simulink model "Drone2_simulink"  (R2024a)
settings: Solver=ode1be  StartTime=0.0  StopTime=1000  FixedStep=0.001  MaxStep=0.001  MinStep=0.00095  RelTol=1e-3
PreLoadFcn:
  | Drone_data;
model workspace: external: MATLAB File C:\Users\admin\OneDrive - Indian Institute of Technology Jodhpur\IIT JODHPUR\Research Work\Amphibious Drone\MATLAB_CODE\2025\New_Drone\Drone_1\Drone1_simulink_DataFile.m (data not in the file)
undefined symbols (not defined in the file): Environment, Newton, Raphson, Vehicle, X, Y, Z
libraries: sm_lib x1684, nesl_utility x63, slpidlib x25, eeGeneralControl x6, matrix_library x3, rllib x2, simulink x2, fl_lib x1, sharedutil x1, SignalEditorBlockLib x1
(part 15 of 17)

== system Drone2_simulink/Physical_system/Drone_Assembly/Cylinder_Assembly/Frontcap/Nut on Cap/Nutwasher_subsystem5 ==
  m3nut1 : sm_lib/Body Elements/File Solid  ExtGeomFileName=socket head cap screw_isM3.STL  UnitType=Custom  ExtGeomFileUnits=mm  StepReaderType=HEX  ExportConvexHullGeometry=off  InertiaType=CalculateFromGeometry  BasedOnType=Density  Density=7800  DensityUnits=kg/m^3  Mass=1  MassUnits=kg  CenterOfMass=[0 0 0]  CenterOfMassUnits=m  MomentsOfInertia=[1 1 1]  MomentsOfInertiaUnits=kg*m^2  ProductsOfInertia=[0 0 0]  ProductsOfInertiaUnits=kg*m^2  GraphicType=FromGeometry  MarkerShape=Sphere  MarkerSize=10  GraphicVisPropType=SimpleVisualProperties  GraphicDiffuseColor=[0.5 0.5 0.5]  GraphicOpacity=1  GraphicSpecularColor=[0.5 0.5 0.5 1.0]  GraphicAmbientColor=[0.15 0.15 0.15 1.0]  GraphicEmissiveColor=[0.0 0.0 0.0 1.0]  GraphicShininess=75  DoExposeReferenceFrame=off  SerializedFrames=<Frames><Frame><Id>Frame1</Id><Value><Name>F1</Name><Origin><Source>CenterOfMassFrame</Source><FeatureName></FeatureName></Origin><PrimaryAxis><DefinedDirection>+Z</DefinedDirection><Source>ReferenceFrame</Source><SourceDirection>-X</SourceDirection><FeatureName></FeatureName></PrimaryAxis><SecondaryAxis><DefinedDirection>+X</DefinedDirection><Source>ReferenceFrame</Source><SourceDirection>+Y</SourceDirection><FeatureName></FeatureName></SecondaryAxis></Value></Frame></Frames>
  m3washer1 : sm_lib/Body Elements/File Solid  ExtGeomFileName=plain washer (type a)_isM3.STL  UnitType=Custom  ExtGeomFileUnits=mm  StepReaderType=HEX  ExportConvexHullGeometry=off  InertiaType=CalculateFromGeometry  BasedOnType=Density  Density=7800  DensityUnits=kg/m^3  Mass=1  MassUnits=kg  CenterOfMass=[0 0 0]  CenterOfMassUnits=m  MomentsOfInertia=[1 1 1]  MomentsOfInertiaUnits=kg*m^2  ProductsOfInertia=[0 0 0]  ProductsOfInertiaUnits=kg*m^2  GraphicType=FromGeometry  MarkerShape=Sphere  MarkerSize=10  GraphicVisPropType=SimpleVisualProperties  GraphicDiffuseColor=[0.5 0.5 0.5]  GraphicOpacity=1  GraphicSpecularColor=[0.5 0.5 0.5 1.0]  GraphicAmbientColor=[0.15 0.15 0.15 1.0]  GraphicEmissiveColor=[0.0 0.0 0.0 1.0]  GraphicShininess=75  DoExposeReferenceFrame=off  SerializedFrames=<Frames><Frame><Id>Frame1</Id><Value><Name>F1</Name><Origin><Source>CenterOfMassFrame</Source><FeatureName></FeatureName></Origin><PrimaryAxis><DefinedDirection>+Z</DefinedDirection><Source>ReferenceFrame</Source><SourceDirection>+Y</SourceDirection><FeatureName></FeatureName></PrimaryAxis><SecondaryAxis><DefinedDirection>+X</DefinedDirection><Source>ReferenceFrame</Source><SourceDirection>+X</SourceDirection><FeatureName></FeatureName></SecondaryAxis></Value></Frame></Frames>
  ofsetfornut : sm_lib/Frames and Transforms/Rigid Transform  RotationMethod=None  FollAlignAxisA=+X  BaseAlignAxisA=+Y  FollAlignAxisB=+Y  BaseAlignAxisB=+Z  RotationStandardAxis=+Z  RotationAngle=180  RotationAngleUnits=deg  RotationArbitraryAxis=[0 0 1]  RotationSequenceAxes=FollowerAxes  RotationSequence=XYX  RotationSequenceAngles=[0 0 0]  RotationSequenceAnglesUnits=deg  RotationMatrix=[1 0 0;0 1 0;0 0 1]  Quaternion=[1 0 0 0]  TranslationMethod=Cartesian  TranslationCartesianOffset=[0 0 -0.0043]  TranslationCartesianOffsetUnits=m  TranslationStandardAxis=+Z  TranslationStandardOffset=0  TranslationStandardOffsetUnits=m  TranslationROffset=0  TranslationROffsetUnits=m  TranslationThetaOffset=0  TranslationThetaOffsetUnits=deg  TranslationZOffset=0  TranslationZOffsetUnits=m
  washercentre to washer1 : sm_lib/Frames and Transforms/Rigid Transform  RotationMethod=None  FollAlignAxisA=+X  BaseAlignAxisA=+Z  FollAlignAxisB=+Y  BaseAlignAxisB=+Y  RotationStandardAxis=+Z  RotationAngle=180  RotationAngleUnits=deg  RotationArbitraryAxis=[0 0 1]  RotationSequenceAxes=FollowerAxes  RotationSequence=XYX  RotationSequenceAngles=[0 0 0]  RotationSequenceAnglesUnits=deg  RotationMatrix=[1 0 0;0 1 0;0 0 1]  Quaternion=[1 0 0 0]  TranslationMethod=Cylindrical  TranslationCartesianOffset=[0.227 0 0]  TranslationCartesianOffsetUnits=m  TranslationStandardAxis=+Z  TranslationStandardOffset=0  TranslationStandardOffsetUnits=m  TranslationROffset=0.0675  TranslationROffsetUnits=m  TranslationThetaOffset=theta  TranslationThetaOffsetUnits=deg  TranslationZOffset=0.00025  TranslationZOffsetUnits=m
  fromcenter : PMIOPort  Side=Left
  connections:
  m3washer1/LConn1 -- washercentre to washer1/RConn1 -- ofsetfornut/LConn1
  ofsetfornut/RConn1 -- m3nut1/LConn1
  fromcenter/RConn1 -- washercentre to washer1/LConn1

== system Drone2_simulink/Physical_system/Drone_Assembly/Cylinder_Assembly/Frontcap/Nut on Cap/Nutwasher_subsystem6 ==
  m3nut1 : sm_lib/Body Elements/File Solid  ExtGeomFileName=socket head cap screw_isM3.STL  UnitType=Custom  ExtGeomFileUnits=mm  StepReaderType=HEX  ExportConvexHullGeometry=off  InertiaType=CalculateFromGeometry  BasedOnType=Density  Density=7800  DensityUnits=kg/m^3  Mass=1  MassUnits=kg  CenterOfMass=[0 0 0]  CenterOfMassUnits=m  MomentsOfInertia=[1 1 1]  MomentsOfInertiaUnits=kg*m^2  ProductsOfInertia=[0 0 0]  ProductsOfInertiaUnits=kg*m^2  GraphicType=FromGeometry  MarkerShape=Sphere  MarkerSize=10  GraphicVisPropType=SimpleVisualProperties  GraphicDiffuseColor=[0.5 0.5 0.5]  GraphicOpacity=1  GraphicSpecularColor=[0.5 0.5 0.5 1.0]  GraphicAmbientColor=[0.15 0.15 0.15 1.0]  GraphicEmissiveColor=[0.0 0.0 0.0 1.0]  GraphicShininess=75  DoExposeReferenceFrame=off  SerializedFrames=<Frames><Frame><Id>Frame1</Id><Value><Name>F1</Name><Origin><Source>CenterOfMassFrame</Source><FeatureName></FeatureName></Origin><PrimaryAxis><DefinedDirection>+Z</DefinedDirection><Source>ReferenceFrame</Source><SourceDirection>-X</SourceDirection><FeatureName></FeatureName></PrimaryAxis><SecondaryAxis><DefinedDirection>+X</DefinedDirection><Source>ReferenceFrame</Source><SourceDirection>+Y</SourceDirection><FeatureName></FeatureName></SecondaryAxis></Value></Frame></Frames>
  m3washer1 : sm_lib/Body Elements/File Solid  ExtGeomFileName=plain washer (type a)_isM3.STL  UnitType=Custom  ExtGeomFileUnits=mm  StepReaderType=HEX  ExportConvexHullGeometry=off  InertiaType=CalculateFromGeometry  BasedOnType=Density  Density=7800  DensityUnits=kg/m^3  Mass=1  MassUnits=kg  CenterOfMass=[0 0 0]  CenterOfMassUnits=m  MomentsOfInertia=[1 1 1]  MomentsOfInertiaUnits=kg*m^2  ProductsOfInertia=[0 0 0]  ProductsOfInertiaUnits=kg*m^2  GraphicType=FromGeometry  MarkerShape=Sphere  MarkerSize=10  GraphicVisPropType=SimpleVisualProperties  GraphicDiffuseColor=[0.5 0.5 0.5]  GraphicOpacity=1  GraphicSpecularColor=[0.5 0.5 0.5 1.0]  GraphicAmbientColor=[0.15 0.15 0.15 1.0]  GraphicEmissiveColor=[0.0 0.0 0.0 1.0]  GraphicShininess=75  DoExposeReferenceFrame=off  SerializedFrames=<Frames><Frame><Id>Frame1</Id><Value><Name>F1</Name><Origin><Source>CenterOfMassFrame</Source><FeatureName></FeatureName></Origin><PrimaryAxis><DefinedDirection>+Z</DefinedDirection><Source>ReferenceFrame</Source><SourceDirection>+Y</SourceDirection><FeatureName></FeatureName></PrimaryAxis><SecondaryAxis><DefinedDirection>+X</DefinedDirection><Source>ReferenceFrame</Source><SourceDirection>+X</SourceDirection><FeatureName></FeatureName></SecondaryAxis></Value></Frame></Frames>
  ofsetfornut : sm_lib/Frames and Transforms/Rigid Transform  RotationMethod=None  FollAlignAxisA=+X  BaseAlignAxisA=+Y  FollAlignAxisB=+Y  BaseAlignAxisB=+Z  RotationStandardAxis=+Z  RotationAngle=180  RotationAngleUnits=deg  RotationArbitraryAxis=[0 0 1]  RotationSequenceAxes=FollowerAxes  RotationSequence=XYX  RotationSequenceAngles=[0 0 0]  RotationSequenceAnglesUnits=deg  RotationMatrix=[1 0 0;0 1 0;0 0 1]  Quaternion=[1 0 0 0]  TranslationMethod=Cartesian  TranslationCartesianOffset=[0 0 -0.0043]  TranslationCartesianOffsetUnits=m  TranslationStandardAxis=+Z  TranslationStandardOffset=0  TranslationStandardOffsetUnits=m  TranslationROffset=0  TranslationROffsetUnits=m  TranslationThetaOffset=0  TranslationThetaOffsetUnits=deg  TranslationZOffset=0  TranslationZOffsetUnits=m
  washercentre to washer1 : sm_lib/Frames and Transforms/Rigid Transform  RotationMethod=None  FollAlignAxisA=+X  BaseAlignAxisA=+Z  FollAlignAxisB=+Y  BaseAlignAxisB=+Y  RotationStandardAxis=+Z  RotationAngle=180  RotationAngleUnits=deg  RotationArbitraryAxis=[0 0 1]  RotationSequenceAxes=FollowerAxes  RotationSequence=XYX  RotationSequenceAngles=[0 0 0]  RotationSequenceAnglesUnits=deg  RotationMatrix=[1 0 0;0 1 0;0 0 1]  Quaternion=[1 0 0 0]  TranslationMethod=Cylindrical  TranslationCartesianOffset=[0.227 0 0]  TranslationCartesianOffsetUnits=m  TranslationStandardAxis=+Z  TranslationStandardOffset=0  TranslationStandardOffsetUnits=m  TranslationROffset=0.0675  TranslationROffsetUnits=m  TranslationThetaOffset=theta  TranslationThetaOffsetUnits=deg  TranslationZOffset=0.00025  TranslationZOffsetUnits=m
  fromcenter : PMIOPort  Side=Left
  connections:
  m3washer1/LConn1 -- washercentre to washer1/RConn1 -- ofsetfornut/LConn1
  ofsetfornut/RConn1 -- m3nut1/LConn1
  fromcenter/RConn1 -- washercentre to washer1/LConn1

== system Drone2_simulink/Physical_system/Drone_Assembly/Cylinder_Assembly/Frontcap/Nut on Cap/Nutwasher_subsystem7 ==
  m3nut1 : sm_lib/Body Elements/File Solid  ExtGeomFileName=socket head cap screw_isM3.STL  UnitType=Custom  ExtGeomFileUnits=mm  StepReaderType=HEX  ExportConvexHullGeometry=off  InertiaType=CalculateFromGeometry  BasedOnType=Density  Density=7800  DensityUnits=kg/m^3  Mass=1  MassUnits=kg  CenterOfMass=[0 0 0]  CenterOfMassUnits=m  MomentsOfInertia=[1 1 1]  MomentsOfInertiaUnits=kg*m^2  ProductsOfInertia=[0 0 0]  ProductsOfInertiaUnits=kg*m^2  GraphicType=FromGeometry  MarkerShape=Sphere  MarkerSize=10  GraphicVisPropType=SimpleVisualProperties  GraphicDiffuseColor=[0.5 0.5 0.5]  GraphicOpacity=1  GraphicSpecularColor=[0.5 0.5 0.5 1.0]  GraphicAmbientColor=[0.15 0.15 0.15 1.0]  GraphicEmissiveColor=[0.0 0.0 0.0 1.0]  GraphicShininess=75  DoExposeReferenceFrame=off  SerializedFrames=<Frames><Frame><Id>Frame1</Id><Value><Name>F1</Name><Origin><Source>CenterOfMassFrame</Source><FeatureName></FeatureName></Origin><PrimaryAxis><DefinedDirection>+Z</DefinedDirection><Source>ReferenceFrame</Source><SourceDirection>-X</SourceDirection><FeatureName></FeatureName></PrimaryAxis><SecondaryAxis><DefinedDirection>+X</DefinedDirection><Source>ReferenceFrame</Source><SourceDirection>+Y</SourceDirection><FeatureName></FeatureName></SecondaryAxis></Value></Frame></Frames>
  m3washer1 : sm_lib/Body Elements/File Solid  ExtGeomFileName=plain washer (type a)_isM3.STL  UnitType=Custom  ExtGeomFileUnits=mm  StepReaderType=HEX  ExportConvexHullGeometry=off  InertiaType=CalculateFromGeometry  BasedOnType=Density  Density=7800  DensityUnits=kg/m^3  Mass=1  MassUnits=kg  CenterOfMass=[0 0 0]  CenterOfMassUnits=m  MomentsOfInertia=[1 1 1]  MomentsOfInertiaUnits=kg*m^2  ProductsOfInertia=[0 0 0]  ProductsOfInertiaUnits=kg*m^2  GraphicType=FromGeometry  MarkerShape=Sphere  MarkerSize=10  GraphicVisPropType=SimpleVisualProperties  GraphicDiffuseColor=[0.5 0.5 0.5]  GraphicOpacity=1  GraphicSpecularColor=[0.5 0.5 0.5 1.0]  GraphicAmbientColor=[0.15 0.15 0.15 1.0]  GraphicEmissiveColor=[0.0 0.0 0.0 1.0]  GraphicShininess=75  DoExposeReferenceFrame=off  SerializedFrames=<Frames><Frame><Id>Frame1</Id><Value><Name>F1</Name><Origin><Source>CenterOfMassFrame</Source><FeatureName></FeatureName></Origin><PrimaryAxis><DefinedDirection>+Z</DefinedDirection><Source>ReferenceFrame</Source><SourceDirection>+Y</SourceDirection><FeatureName></FeatureName></PrimaryAxis><SecondaryAxis><DefinedDirection>+X</DefinedDirection><Source>ReferenceFrame</Source><SourceDirection>+X</SourceDirection><FeatureName></FeatureName></SecondaryAxis></Value></Frame></Frames>
  ofsetfornut : sm_lib/Frames and Transforms/Rigid Transform  RotationMethod=None  FollAlignAxisA=+X  BaseAlignAxisA=+Y  FollAlignAxisB=+Y  BaseAlignAxisB=+Z  RotationStandardAxis=+Z  RotationAngle=180  RotationAngleUnits=deg  RotationArbitraryAxis=[0 0 1]  RotationSequenceAxes=FollowerAxes  RotationSequence=XYX  RotationSequenceAngles=[0 0 0]  RotationSequenceAnglesUnits=deg  RotationMatrix=[1 0 0;0 1 0;0 0 1]  Quaternion=[1 0 0 0]  TranslationMethod=Cartesian  TranslationCartesianOffset=[0 0 -0.0043]  TranslationCartesianOffsetUnits=m  TranslationStandardAxis=+Z  TranslationStandardOffset=0  TranslationStandardOffsetUnits=m  TranslationROffset=0  TranslationROffsetUnits=m  TranslationThetaOffset=0  TranslationThetaOffsetUnits=deg  TranslationZOffset=0  TranslationZOffsetUnits=m
  washercentre to washer1 : sm_lib/Frames and Transforms/Rigid Transform  RotationMethod=None  FollAlignAxisA=+X  BaseAlignAxisA=+Z  FollAlignAxisB=+Y  BaseAlignAxisB=+Y  RotationStandardAxis=+Z  RotationAngle=180  RotationAngleUnits=deg  RotationArbitraryAxis=[0 0 1]  RotationSequenceAxes=FollowerAxes  RotationSequence=XYX  RotationSequenceAngles=[0 0 0]  RotationSequenceAnglesUnits=deg  RotationMatrix=[1 0 0;0 1 0;0 0 1]  Quaternion=[1 0 0 0]  TranslationMethod=Cylindrical  TranslationCartesianOffset=[0.227 0 0]  TranslationCartesianOffsetUnits=m  TranslationStandardAxis=+Z  TranslationStandardOffset=0  TranslationStandardOffsetUnits=m  TranslationROffset=0.0675  TranslationROffsetUnits=m  TranslationThetaOffset=theta  TranslationThetaOffsetUnits=deg  TranslationZOffset=0.00025  TranslationZOffsetUnits=m
  fromcenter : PMIOPort  Side=Left
  connections:
  m3washer1/LConn1 -- washercentre to washer1/RConn1 -- ofsetfornut/LConn1
  ofsetfornut/RConn1 -- m3nut1/LConn1
  fromcenter/RConn1 -- washercentre to washer1/LConn1

== matlab function Drone2_simulink/Controller/Aerial_control/Aerial Control ==
  data: Thrust input; FRF output; TRF output; Roll input; Pitch input; Yaw input; FRB output; TRB output; FLF output; TLF output; FLB output; TLB output; k parameter; Zd input; Z input; ez input; ez_dot input; er input; er_dot input; ep input; ep_dot input; eyaw input; eyaw_dot input; Max_thrust parameter; Min_torque parameter; Max_torque parameter; Min_Dthrust parameter; dt parameter; EZ_DB parameter; ER_DB parameter; EP_DB parameter; Eyaw_DB parameter
function [FRF,TRF, FRB, TRB,FLF,TLF, FLB,TLB] = fcn(Thrust,Roll,Pitch,Yaw,k,Zd,Z,ez,ez_dot,er,er_dot,ep,ep_dot,eyaw,eyaw_dot, Max_thrust, Min_torque, Max_torque,Min_Dthrust,dt,EZ_DB, ER_DB, EP_DB, Eyaw_DB)
A  = [1 1 1 1;0.276 0.276 -0.276 -0.276;-0.1575 0.1825 0.1825 -0.1575;-k k -k k];
if Zd<=0 && Z >=0
   [FRF, FRB,FLF, FLB] = deal(0);
   [TRF, TRB,TLF,TLB] = deal(0);
    return
elseif Zd<=0 && Z<0
    [FRF,TRF, FRB, TRB,FLF,TLF, FLB,TLB] = deal(0);
    return
elseif Z <=-0.15
    [FRF,TRF, FRB, TRB,FLF,TLF, FLB,TLB] = deal(0);
    return
end


Force = A\[Thrust;Roll;Pitch;Yaw];



%% Adaptive Part
K_TRIM = 0.002;
K_RATE = 0.005;

adapt_gateZ = 1.0 / (1.0 + K_RATE*abs(ez_dot));     % suppress when moving fast
if abs(ez) < EZ_DB
    adapt_gateZ = 0.25 * adapt_gateZ;                 % slower inside small band0.2
end
dSum_trimZ = K_TRIM * ez * adapt_gateZ;  

adapt_gateR = 1.0 / (1.0 + K_RATE*abs(er_dot));     % suppress when moving fast
if abs(er) < ER_DB
    adapt_gateR = 0.25* adapt_gateR;                 % slower inside small band0.2
end
dSum_trimR = K_TRIM * ez * adapt_gateR; 

adapt_gateP = 1.0 / (1.0 + K_RATE*abs(ep_dot));     % suppress when moving fast
if abs(ep) < EP_DB
    adapt_gateP = 0.25 * adapt_gateP;                 % slower inside small band0.2
end
dSum_trimP = K_TRIM * ez * adapt_gateP;  

adapt_gateY = 1.0 / (1.0 + K_RATE*abs(eyaw_dot));     % suppress when moving fast
if abs(eyaw) < Eyaw_DB
    adapt_gateY = 0.25 * adapt_gateY;                 % slower inside small band0.2
end
dSum_trimY = K_TRIM * ez * adapt_gateY;  

FLF = Force(1);%+dSum_trimZ*dt+dSum_trimR*dt-dSum_trimP*dt ;
FLB = Force(2);%+dSum_trimZ*dt+dSum_trimR*dt+dSum_trimP*dt;
FRB = Force(3);%+dSum_trimZ*dt-dSum_trimR*dt+dSum_trimP*dt;
FRF = Force(4);%+dSum_trimZ*dt-dSum_trimR*dt-dSum_trimP*dt;
TRF = k*FRF;%+dSum_trimY;
TRB = k*FRB;%-dSum_trimY;
TLF = k*FLF;%-dSum_trimY;
TLB = k*FLB;%+dSum_trimY;

FLF = clamp(FLF,Min_Dthrust,Max_thrust);
FLB = clamp(FLB,Min_Dthrust,Max_thrust);
FRF = clamp(FRF,Min_Dthrust,Max_thrust);
FRB = clamp(FRB,Min_Dthrust,Max_thrust);

TLF = clamp(TLF,Min_torque,Max_torque);
TLB = clamp(TLB,Min_torque,Max_torque);
TRF = clamp(TRF,Min_torque,Max_torque);
TRB = clamp(TRB,Min_torque,Max_torque);
end


function y = clamp(x, xmin, xmax)
    y = min(max(x, xmin), xmax);
end

== matlab function Drone2_simulink/Controller/RL System/MATLAB Function2 ==
  data: Obsevation input; reward output; Desired input; feedback input; Const parameter
%% reward Function
function reward = rewardFunction(Obsevation,Desired,feedback, Const)
% Target depth and pitch
depth = Observation(1);
depthRate = Obsevation(2);
pitch= Obsevation(3);
pitchRate = Obsevation(4);
Fs1pos = Obsevation(5);
Fs2pos = Obsevation(6);
Fs1vel = Obsevation(7);
Fs2vel = Obsevation(8);
Bspos = Obsevation(9);
Bsvel = Obsevation(10);
A = const;
depth_ref = Desired(1);
pitch_ref = Desired(2);



depth_error = depth - depth_ref;
pitch_error = pitch - pitch_ref;


reward = - (5 * depth_error^2 + 2 * pitch_error^2 + 0.5 * depthRate^2 + 0.5 * pitchRate^2);
end

== matlab function Drone2_simulink/Controller/RL System/MATLAB Function3 ==
  data: Observation input; reward output; Desired input; MaxVel parameter; MaxPose parameter; MinPose parameter; Delta parameter; K parameter
%% reward Function
function reward = rewardFunction(Observation,Desired, MaxVel, MaxPose, MinPose, Delta, K)
% Target depth and pitch
depth = Observation(1);
depthRate = Observation(2);
pitch= Observation(3);
pitchRate = Observation(4);
Fs1pos = Observation(5);
Fs2pos = Observation(6);
Fs1vel = Observation(7);
Fs2vel = Observation(8);
Bspos = Observation(9);
Bsvel = Observation(10);


Syring1Reward = syringeRewardSigmoid(Fs1pos,Fs1vel,MinPose,MaxPose,Delta,MaxVel,K);
Syring2Reward = syringeRewardSigmoid(Fs2pos,Fs2vel,MinPose,MaxPose,Delta,MaxVel,K);
Syring3Reward = syringeRewardSigmoid(Bspos,Bsvel,MinPose,MaxPose,Delta,MaxVel,K);


depth_ref = Desired(1);
pitch_ref = Desired(2);



depth_error = depth - depth_ref;
pitch_error = pitch - pitch_ref;


reward = - (5 * depth_error^2 + 0.1 * pitch_error^2 + 0.25 * depthRate^2 + 0.5 * pitchRate^2+0.25*depth_error*depthRate+0.25*pitchRate*pitch_error+depth_error*((Fs1vel+Fs2vel)/2+Bsvel)) + 02*(Syring1Reward+Syring2Reward+Syring3Reward);
end


function reward = syringeRewardSigmoid(pos, vel, minPos, maxPos, delta, vmax, k)
    % Position penalty
    p1 = 1 / (1 + exp(-k * (pos - (maxPos - delta))));
    p2 = 1 / (1 + exp(k  * (pos - (minPos + delta))));
    penalty_pos = p1 + p2;

    % Velocity penalty
    penalty_vel = 1 / (1 + exp(-k * (abs(vel) - vmax)));

    % Total penalty
    total_penalty = penalty_pos + 1.2*penalty_vel;

    % Reward is negative penalty
    reward = -total_penalty;
end

== matlab function Drone2_simulink/Controller/RL System/MATLAB Function4 ==
  data: obs input; reward output; desired input; MaxVel parameter; MaxPose parameter; MinPose parameter; Delta parameter
%% reward Function
%function reward = rewardFunction(Observation,Desired, MaxVel, MaxPose, MinPose, Delta, K)


function reward = smoothReward(obs, desired,MaxVel, MaxPose, MinPose, Delta)

    % Unpack observations
    z           = obs(1);    % depth
    z_dot       = obs(2);    % vertical speed
    pitch       = obs(3);    % pitch
    pitch_dot   = obs(4);    % pitch rate
    syrPosFL     = obs(5);    % front syringe position
    syrVelFL     = obs(6);    % front syringe velocity
    syrPosFR     = obs(7);    % back syringe position
    syrVelFR     = obs(8);    % back syringe velocity
    syrPosB     = obs(9);    % back syringe position
    syrVelB    = obs(10);    % back syringe velocity
    syrPosF = (syrPosFR+syrPosFL)/2;
    syrVelF= (syrVelFL+syrVelFR)/2;

    % Desired states
    z_des       = desired(1);
    pitch_des   = desired(2);

    % Errors
    err_z       = z-z_des;
    err_pitch   = pitch - pitch_des;

    % --- Smooth reward components ---

    % 1. Penalize total absolute error
    reward_err = - 0.5*(abs(err_z) + 0.025 * abs(err_pitch));

    % 2. Encourage corrective motion (dot product of error and velocity)
    reward_z_dot      = -0.05 * tanh(err_z * z_dot);
    reward_pitch_dot  = -0.005 * tanh(err_pitch * pitch_dot);

    % 3. Encourage syringe motion that helps depth correction
    reward_syringe_dir =  0.01*tanh(err_z * (syrVelF + syrVelB));

    % 4. Penalize being near limits of syringe stroke (soft cushion)
    minPos = MinPose; maxPos = MaxPose; cushion = Delta;

    penalty_cushionF = -0.05 * exp( - ((syrPosF - (minPos + cushion)) * (maxPos - cushion - syrPosF)) * 1e2 );
    penalty_cushionB = -0.05 * exp( - ((syrPosB - (minPos + cushion)) * (maxPos - cushion - syrPosB)) * 1e2 );

    % 5. Penalize excessive syringe velocity (soft)
    maxVel = MaxVel;
    penalty_velF = -0.1 * max(0, abs(syrVelF) - maxVel);
    penalty_velB = -0.1 * max(0, abs(syrVelB) - maxVel);

    % Final reward
    reward = reward_err + reward_z_dot + reward_pitch_dot + ...
             reward_syringe_dir + ...
             penalty_cushionF + penalty_cushionB + ...
             penalty_velF + penalty_velB;

end



% function reward = syringeRewardSigmoid(pos, vel, minPos, maxPos, delta, vmax, k)
%     % Position penalty
%     p1 = 1 / (1 + exp(-k * (pos - (maxPos - delta))));
%     p2 = 1 / (1 + exp(k  * (pos - (minPos + delta))));
%     penalty_pos = p1 + p2;
% 
%     % Velocity penalty
%     penalty_vel = 1 / (1 + exp(-k * (abs(vel) - vmax)));
% 
%     % Total penalty
%     total_penalty = penalty_pos + 1.2*penalty_vel;
% 
%     % Reward is negative penalty
%     reward = -total_penalty;
% end

== matlab function Drone2_simulink/Controller/Underwater_Syringe_Actuation/MATLAB Function7 ==
  settings: updateMethod=DISCRETE
  data: Z_desired input; Z input; F_b input; tb input; Vf_cmd output; ez input; ez_dot input; etheta input; etheta_dot input; Vb_cmd output; Vf_prev input; Vb_prev input; Vf_trim_hat output; Vb_trim_hat output; Max parameter; Min parameter; DFRate parameter; DMRate parameter; DSRate parameter; Dpanelty parameter; EZDB parameter; PLRate parameter; PKRate parameter; ETDB parameter; RHO parameter; G parameter; AS parameter; HF parameter; DT parameter
function [Vf_cmd, Vb_cmd, Vf_trim_hat, Vb_trim_hat]= ...
    syringe_allocation_adaptive(Z_desired, Z,F_b,tb, ez, ez_dot,etheta,etheta_dot,Vf_prev, Vb_prev,Max, Min,DFRate, DMRate, DSRate, Dpanelty, EZDB, PLRate, PKRate, ETDB,RHO, G,AS,HF,DT)
% Depth-only allocator with adaptive trims for 2 front syringes (identical) + 1 rear.
% Units: meters of stroke for all volumes/positions.
% Outputs:
%   Vf_cmd       -> per-front syringe command (send same to both fronts)
%   Vb_cmd       -> rear syringe command
%   Vf_trim_hat  -> current estimated per-front trim (for datalogging/observability)
%   Vb_trim_hat  -> current estimated rear trim

% -------- Tunables --------
rho = RHO; %1000;         % kg/m^3
g   = G; %9.81;         % m/s^2
A   = AS; %0.026;        % m^2  (verify; adjust to your syringe)
l= HF; %0.2;
V_MIN = Min;      % m (5 mm)
V_MAX = Max;      % m (100 mm)
V_DOT_MAX = 0.012;  % m/s (12 mm/s)
dt = DT; %0.001;
tb = clamp(tb,-5,5);

% -------- Persistent state for trim estimates --------
persistent VF_TRIM VF_TRIM_INIT VB_TRIM VB_TRIM_INIT inited
if isempty(inited)
    VF_TRIM_INIT = 0.046;   % m  (assumed 46 mm per front syringe)
    VB_TRIM_INIT = 0.031;   % m  (assumed 31 mm rear syringe)
    VF_TRIM = VF_TRIM_INIT;
    VB_TRIM = VB_TRIM_INIT;
    inited = true;
end


if Z_desired >-0.1 || Z>=0
    Vf_cmd = Min;
    Vb_cmd = Min;
    Vf_trim_hat = Vf_cmd;
    Vb_trim_hat = Vb_cmd;
    return
end


persistent t
if isempty(t)
    t =0;
end

% S = 2*Vf_prev+Vb_prev;
 % kp =0;
% Adaptive-trim gains (start small)
if abs(ez) > 1
    K_TRIM_eff = DFRate;%0.02;   % fast learning when far
    kp = 0;
elseif abs(ez) > 0.6
    K_TRIM_eff = DMRate; %0.005;   % medium
    kp= 0;
else
    K_TRIM_eff = DSRate; %0.002;  % fine adjust near trim
    if abs(ez)<0.2
        t=t+1;
    else
        t = 0;
    end
    if t>50000
        kp=1;
    else
        kp =0;
    end

end


K_TRIM  =K_TRIM_eff;    % (m/s per m of depth error)  VERY SLOW 0.002
K_RATE  = Dpanelty; %0.05;     % dimensionless; reduces adaptation if |ez_dot| is large 0.05
EZ_DB   = EZDB; %0.05;     % m; within 10 cm, adapt 5x slower to avoid chatter 0.05

KP_TRIM  =PLRate; %0.0002;    % (m/s per m of depth error)  VERY SLOW 0.002
K_Pitch_Rate  = PKRate; %0.05;     % dimensionless; reduces adaptation if |ez_dot| is large 0.05
Etheta_DB   = deg2rad(ETDB); %pi/60;     % m; within 10 cm, adapt 5x slower to avoid chatter 0.05




% -------- Fast (reactive) path from F_b to stroke increments --------
% F_b = rho*g*A*(2*Vf_inc + Vb_inc)
dSum = F_b / (rho*g*A);   % meters of stroke-sum (2*Vf + Vb)
Vf_inc_fast = 0.25 * dSum;  % per front syringe
Vb_inc_fast = 0.50 * dSum;  % rear


%-------- Pitch Control-----
mSum = tb/(rho*g*A*l);
%mSum = tb/(rho*g*A*(2*(l-0.5*Vf_prev)-(l-0.5*Vb_prev)));
%mSum = (tb-rho*A*g*S*(l-0.5*Vf_prev))/(rho*g*A*(2*(l-0.5*Vf_prev)-(l-0.5*Vb_prev)));
Vf_inc_pitch = 0.5*mSum;
vb_inc_pitch = -0.5*mSum;
Vf_inc_pitch = clamp(Vf_inc_pitch,-0.005,0.005);
vb_inc_pitch = clamp(vb_inc_pitch,-0.01,0.01);


% -------- Slow (adaptive) trim update to remove drift --------
% adapt_gate = exp(-K_RATE*abs(ez_dot));

adapt_gate = 1.0 / (1.0 + K_RATE*abs(ez_dot));     % suppress when moving fast
if abs(ez) < EZ_DB
    adapt_gate = 0.25 * adapt_gate;                 % slower inside small band0.2
end
dSum_trim = K_TRIM * ez * adapt_gate;              % m/s equivalent stroke-sum


%------ Pitch updates

pitch_gate = kp/(1.0+K_Pitch_Rate*abs(etheta_dot));
if abs(etheta) <Etheta_DB
    pitch_gate = 0.2*pitch_gate;
end
mSum_trim = KP_TRIM*etheta*pitch_gate;
mSum_trim = clamp(mSum_trim,-0.01,0.01);


Vf_trim_update = 0.25 * dSum_trim * dt-0.25*mSum_trim*dt;            % per front syringe
Vb_trim_update = 0.50 * dSum_trim * dt+0.50*mSum_trim*dt;            % rear

VF_TRIM = clamp(VF_TRIM + Vf_trim_update, V_MIN, V_MAX);
VB_TRIM = clamp(VB_TRIM + Vb_trim_update, V_MIN, V_MAX);

% -------- Combine trim + fast correction --------
Vf_target = VF_TRIM + Vf_inc_fast+0*kp*Vf_inc_pitch;
Vb_target = VB_TRIM + Vb_inc_fast+0*kp*vb_inc_pitch;

% -------- Stroke clamp --------
Vf_target = clamp(Vf_target, V_MIN, V_MAX);
Vb_target = clamp(Vb_target, V_MIN, V_MAX);
Vf_cmd = Vf_target;
Vb_cmd = Vb_target;
% % -------- Rate limit (12 mm/s) --------
% Vf_cmd = rate_limit(Vf_target, Vf_prev, V_DOT_MAX, dt);
% Vb_cmd = rate_limit(Vb_target, Vb_prev, V_DOT_MAX, dt);

% Expose trims for logging/next block
Vf_trim_hat = VF_TRIM;
Vb_trim_hat = VB_TRIM;

end

% ===== helpers =====
function y = clamp(x, xmin, xmax)
    y = min(max(x, xmin), xmax);
end

% function y = rate_limit(cmd, prev, vdot_max, dt)
%     max_step = vdot_max * max(dt,1e-4);
%     y = clamp(cmd, prev - max_step, prev + max_step);
% end

== matlab function Drone2_simulink/Controller/Commented functions/MATLAB Function8 ==
  settings: updateMethod=DISCRETE
  data: F_b input; Vf_cmd output; ez input; ez_dot input; Vb_cmd output; Vf_prev input; Vb_prev input; Vf_trim_hat output; Vb_trim_hat output
function [Vf_cmd, Vb_cmd, Vf_trim_hat, Vb_trim_hat]= ...
    syringe_allocation_adaptive(F_b, ez, ez_dot, Vf_prev, Vb_prev)
% Depth-only allocator with adaptive trims for 2 front syringes (identical) + 1 rear.
% Units: meters of stroke for all volumes/positions.
% Outputs:
%   Vf_cmd       -> per-front syringe command (send same to both fronts)
%   Vb_cmd       -> rear syringe command
%   Vf_trim_hat  -> current estimated per-front trim (for datalogging/observability)
%   Vb_trim_hat  -> current estimated rear trim

% -------- Tunables --------
rho = 1000;         % kg/m^3
g   = 9.81;         % m/s^2
A   = 0.026;        % m^2  (verify; adjust to your syringe)
V_MIN = 0.005;      % m (5 mm)
V_MAX = 0.1;      % m (100 mm)
V_DOT_MAX = 0.012;  % m/s (12 mm/s)
dt = 0.001;
% Adaptive-trim gains (start small)
if abs(ez) > 0.1
    K_TRIM_eff = 0.05;   % fast learning when far
elseif abs(ez) > 0.02
    K_TRIM_eff = 0.01;   % medium
else
    K_TRIM_eff = 0.002;  % fine adjust near trim
end


K_TRIM  =0.002;    % (m/s per m of depth error)  VERY SLOW 0.002
K_RATE  = 0.05;     % dimensionless; reduces adaptation if |ez_dot| is large 0.05
EZ_DB   = 0.05;     % m; within 1 cm, adapt 5x slower to avoid chatter 0.05

% -------- Persistent state for trim estimates --------
persistent VF_TRIM VF_TRIM_INIT VB_TRIM VB_TRIM_INIT inited
if isempty(inited)
    VF_TRIM_INIT = 0.046;   % m  (assumed 46 mm per front syringe)
    VB_TRIM_INIT = 0.031;   % m  (assumed 31 mm rear syringe)
    VF_TRIM = VF_TRIM_INIT;
    VB_TRIM = VB_TRIM_INIT;
    inited = true;
end

% -------- Fast (reactive) path from F_b to stroke increments --------
% F_b = rho*g*A*(2*Vf_inc + Vb_inc)
dSum = F_b / (rho*g*A);   % meters of stroke-sum (2*Vf + Vb)
Vf_inc_fast = 0.25 * dSum;  % per front syringe
Vb_inc_fast = 0.50 * dSum;  % rear

% -------- Slow (adaptive) trim update to remove drift --------
% adapt_gate = exp(-K_RATE*abs(ez_dot));

adapt_gate = 1.0 / (1.0 + K_RATE*abs(ez_dot));     % suppress when moving fast
if abs(ez) < EZ_DB
    adapt_gate = 0.25 * adapt_gate;                 % slower inside small band0.2
end
dSum_trim = K_TRIM * ez * adapt_gate;              % m/s equivalent stroke-sum
Vf_trim_update = 0.25 * dSum_trim * dt;            % per front syringe
Vb_trim_update = 0.50 * dSum_trim * dt;            % rear

VF_TRIM = clamp(VF_TRIM + Vf_trim_update, V_MIN, V_MAX);
VB_TRIM = clamp(VB_TRIM + Vb_trim_update, V_MIN, V_MAX);

% -------- Combine trim + fast correction --------
Vf_target = VF_TRIM + Vf_inc_fast;
Vb_target = VB_TRIM + Vb_inc_fast;

% -------- Stroke clamp --------
Vf_target = clamp(Vf_target, V_MIN, V_MAX);
Vb_target = clamp(Vb_target, V_MIN, V_MAX);
Vf_cmd = Vf_target;
Vb_cmd = Vb_target;
% % -------- Rate limit (12 mm/s) --------
% Vf_cmd = rate_limit(Vf_target, Vf_prev, V_DOT_MAX, dt);
% Vb_cmd = rate_limit(Vb_target, Vb_prev, V_DOT_MAX, dt);

% Expose trims for logging/next block
Vf_trim_hat = VF_TRIM;
Vb_trim_hat = VB_TRIM;

end

% ===== helpers =====
function y = clamp(x, xmin, xmax)
    y = min(max(x, xmin), xmax);
end

function y = rate_limit(cmd, prev, vdot_max, dt)
    max_step = vdot_max * max(dt,1e-4);
    y = clamp(cmd, prev - max_step, prev + max_step);
end

== matlab function Drone2_simulink/Controller/Commented functions/MATLAB Function5 ==
  data: Z input; FS output; Pitch input; BS output; Max parameter; Min parameter; density input; syringe_area input; gravity input
function [FS,BS] = fcn(Z,Pitch,Max, Min,density,syringe_area,gravity)


%#codegen
C = density*syringe_area*gravity;
H = Z/C;
syms x_f
x_b = H-2*x_f;
f= (2*l*x_f-(x_f^2))-(l*x_b-(x_b^2));
eqn = f == Pitch/C;

sol = double(solve(eqn,x_f));
solb = H-2.*sol;
end

== matlab function Drone2_simulink/Controller/Commented functions/MATLAB Function6 ==
  data: F_b input; Vf output; tau input; Vb output; Vf_prev input; Vb_prev input
function [Vf, Vb] = syringe_allocation(F_b, tau, Vf_prev, Vb_prev)
% Inputs:
%   F_b     -> required buoyancy force from depth PID
%   tau     -> required pitch torque from pitch PD
%   Vf_prev -> previous front syringe volume (mm)
%   Vb_prev -> previous back syringe volume (mm)
%   dt      -> sample time (s)

% Parameters
rho = 1000;       % water density (kg/m^3)
g   = 9.81;
A   = 0.026;       % syringe piston area (m^2) -> adjust for your syringe
l   = 0.2;        % lever arm distance (m)
Vmin = 0.005; Vmax = 0.1;  % m stroke
Vdot_max = 0.012;
dt = 0.001;
%% Depth control contribution
dV_depth = F_b / (rho * g * A ); % in m (all syringes share)
Vf_depth = dV_depth/4;
Vb_depth = dV_depth/2;

%% Pitch control contribution
dV_pitch = tau / (rho * g * l * A ); % m equivalent
Vf_pitch = dV_pitch/2;
Vb_pitch = -dV_pitch;

%% Combine contributions
Vf = Vf_prev +(Vf_depth); 
Vb = Vb_prev + (Vb_depth);

%% Apply limits (stroke and speed)
% Clamp by stroke
Vf = min(max(Vf, Vmin), Vmax);
Vb = min(max(Vb, Vmin), Vmax);

% Clamp by speed
% Vf = min(max(Vf, Vf_prev - Vdot_max*dt), Vf_prev + Vdot_max*dt);
% Vb = min(max(Vb, Vb_prev - Vdot_max*dt), Vb_prev + Vdot_max*dt);

end

== matlab function Drone2_simulink/Controller/Underwater_Syringe_Actuation/MATLAB Function1 ==
  settings: updateMethod=DISCRETE
  data: F_b input; Z input; Zdesired input; ez input; ez_dot input; dt parameter; rho parameter; A parameter; Vf_cmd output; Vb_cmd output; Vf_trim_hat output; Vb_trim_hat output; g parameter; V_MAX parameter; V_MIN parameter; V_DOT_MAX parameter; Kp_pos parameter; Kp_vel parameter; Ez_high parameter; Kr parameter; sigma parameter
function [Vf_cmd, Vb_cmd, Vf_trim_hat, Vb_trim_hat] = ...
    syringe_allocation_adaptive_3(F_b, Z,Zdesired,ez, ez_dot, dt,rho,A,g, V_MAX, V_MIN, V_DOT_MAX, Kp_pos, Kp_vel, Ez_high, Kr, sigma)
%#codegen
% Adaptive allocation for 2-front + 1-rear syringes
% Implements depth-priority control with sigma-region energy saving
% Author: Shrivi Jay Khatri

%% --- Physical Parameters ---
% rho = 1000;     % kg/m^3
% g   = 9.81;     % m/s^2
% A   = 0.026;    % m^2 (syringe cross-section area)
% V_MIN = 0.005;  % m
% V_MAX = 0.100;  % m
% V_DOT_MAX = 0.012; % m/s (12 mm/s)
% 
% %% --- Adaptive Tuning Parameters ---
% Kp_pos = 0.25;     % proportional position gain
% Kp_vel = 0.02;     % velocity-region damping gain
% Kr     = 2.0;      % rate sensitivity (adaptive damping)
% sigma  = 0.01;     % deadband threshold (m)
% Ez_high = 0.05;    % large-error boundary (m)

%% --- Persistent Adaptive Trims ---
persistent Vf_trim Vb_trim inited
if isempty(inited)
    Vf_trim = 0.046;   % Initial trim (front, m)
    Vb_trim = 0.031;   % Initial trim (rear, m)
    inited = true;
end
if Zdesired>=0.1 || Z>0
    Vf_cmd= V_MIN;
    Vf_trim_hat = V_MIN;
    Vb_cmd = V_MIN;
    Vb_trim_hat =V_MIN;
    return
end
%% --- Compute Effective Stroke Change from Force Demand ---
dSum = F_b / (rho * g * A);   % Total stroke equivalent (2Vf + Vb)
Vf_inc = 0.25 * dSum;         % each front syringe increment
Vb_inc = 0.50 * dSum;         % rear syringe increment

%% --- Adaptive Trim Update Logic ---
if abs(ez) > Ez_high
    % Region 1: Large error → aggressive move
    dVf_trim = sign(ez) * V_DOT_MAX * dt * 0.8;
    dVb_trim = sign(ez) * V_DOT_MAX * dt * 0.8;

elseif abs(ez) > sigma
    % Region 2: Moderate error → position-based slow adaptation
    adapt_factor = 1 / (1 + Kr * abs(ez_dot));
    dSum_trim = Kp_pos * ez * adapt_factor * dt;
    dVf_trim = 0.25 * dSum_trim;
    dVb_trim = 0.50 * dSum_trim;

else
    % Region 3: Small error → velocity-based energy saving
    adapt_factor = 1 / (1 + Kr * abs(ez_dot));
    dSum_trim = -Kp_vel * ez_dot * adapt_factor * dt;
    dVf_trim = 0.25 * dSum_trim;
    dVb_trim = 0.50 * dSum_trim;
end

%% --- Update and Clamp Trims ---
Vf_trim = clamp(Vf_trim + dVf_trim, V_MIN, V_MAX);
Vb_trim = clamp(Vb_trim + dVb_trim, V_MIN, V_MAX);

%% --- Combine Trim and Fast Correction ---
Vf_target = Vf_trim + Vf_inc;
Vb_target = Vb_trim + Vb_inc;

%% --- Clamp Syringe Limits ---
Vf_cmd = clamp(Vf_target, V_MIN, V_MAX);
Vb_cmd = clamp(Vb_target, V_MIN, V_MAX);

%% --- Outputs for Observation ---
Vf_trim_hat = Vf_trim;
Vb_trim_hat = Vb_trim;

end

%% === Helper Functions ===
function y = clamp(x, xmin, xmax)
    y = min(max(x, xmin), xmax);
end
